simulink model "HW2_CTD_system_Based_TF2"  (R2015a)
settings: Solver=ode45  StartTime=0.0  StopTime=10.0  RelTol=1e-3
values from neighbouring files (symbols this model uses):
  A = [0 1;-3 -2]    [HW2.m]    (also in HW2_revised.m)
  B = [0; 1]    [HW2.m]    (also in HW2_revised.m)
  C = [1 1]    [HW2.m]    (also in HW2_revised.m)
  Gamma_0 = (real(G^(1/3))-eye(n))*inv(A)*B    [HW2.m]    (also in HW2_revised.m = (real(G^(1-simDelay/Ts))-eye(n))*inv(A)*B)
  Gamma_1 = (G-real(G^(1/3)))*inv(A)*B    [HW2.m]    (also in HW2_revised.m = (G-real(G^(1-simDelay/Ts)))*inv(A)*B)
  simDelay = delay_time    [HW2_revised.m]
  Tf = 0.06    [HW2.m]    (also in HW2_revised.m)
undefined symbols (not defined in the file or in its folder): G
libraries: cstblocks x1
settings Model: Creator=123  LastModifiedBy=123

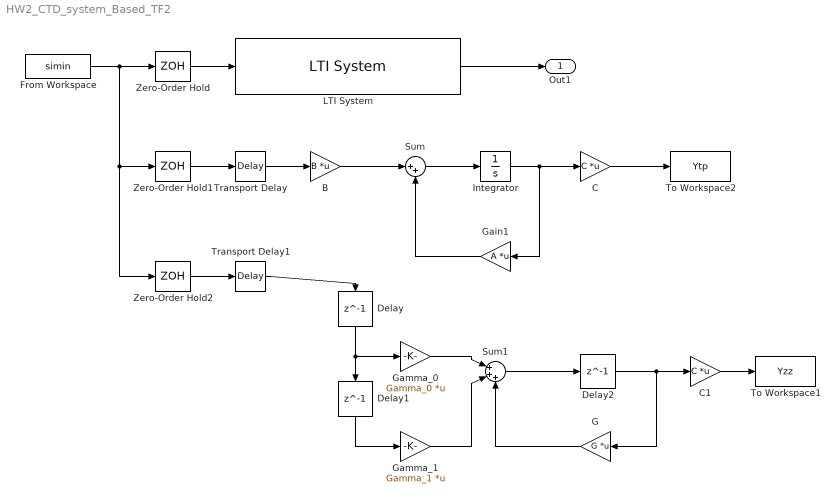
== system HW2_CTD_system_Based_TF2 ==
  B : Gain  Gain=B  Multiplication=Matrix(K*u)
  C : Gain  Gain=C  Multiplication=Matrix(K*u)
  C1 : Gain  Gain=C  Multiplication=Matrix(K*u)
  Delay : Delay  DelayLength=1  InitialCondition=0  SampleTime=Tf
  Delay1 : Delay  DelayLength=1  InitialCondition=0  SampleTime=Tf
  Delay2 : Delay  DelayLength=1  InitialCondition=0  SampleTime=Tf
  From Workspace : FromWorkspace  VariableName=simin  SampleTime=0
  G : Gain  Gain=G  Multiplication=Matrix(K*u)
  Gain1 : Gain  Gain=A  Multiplication=Matrix(K*u)
  Gamma_0 : Gain  Gain=Gamma_0  Multiplication=Matrix(K*u)
  Gamma_1 : Gain  Gain=Gamma_1  Multiplication=Matrix(K*u)
  Integrator : Integrator
  LTI System : cstblocks/LTI System  sys=ss(A,B,C,0,'InputDelay',simDelay)  IC=[0 0]
  Sum : Sum  Inputs=|++
  Sum1 : Sum  Inputs=|+++
  To Workspace1 : ToWorkspace  VariableName=Yzz  SampleTime=-1
  To Workspace2 : ToWorkspace  VariableName=Ytp  SampleTime=-1
  Transport Delay : TransportDelay  DelayTime=simDelay
  Transport Delay1 : TransportDelay  DelayTime=simDelay
  Zero-Order Hold : ZeroOrderHold  SampleTime=Tf
  Zero-Order Hold1 : ZeroOrderHold  SampleTime=Tf
  Zero-Order Hold2 : ZeroOrderHold  SampleTime=Tf
  Out1 : Outport
  wires:
  From Workspace/1 -> Zero-Order Hold2/1, Zero-Order Hold1/1, Zero-Order Hold/1
  LTI System/1 -> Out1/1
  Zero-Order Hold/1 -> LTI System/1
  Zero-Order Hold1/1 -> Transport Delay/1
  Transport Delay/1 -> B/1
  B/1 -> Sum/1
  Sum/1 -> Integrator/1
  Gain1/1 -> Sum/2
  Integrator/1 -> C/1, Gain1/1
  Delay/1 -> Gamma_0/1, Delay1/1
  Delay1/1 -> Gamma_1/1
  Gamma_0/1 -> Sum1/1
  Gamma_1/1 -> Sum1/2
  Sum1/1 -> Delay2/1
  Delay2/1 -> C1/1, G/1
  G/1 -> Sum1/3
  C/1 -> To Workspace2/1
  C1/1 -> To Workspace1/1
  Transport Delay1/1 -> Delay/1
  Zero-Order Hold2/1 -> Transport Delay1/1
